simulink model "BBB_Gyro_Test_SFunction_Mask"  (R2013a)
settings: Solver=FixedStepDiscrete  StartTime=0.0  StopTime=inf  FixedStep=0.01  RelTol=1e-3
settings Model: SimulationMode=external  ExtModeTrigDuration=100  Creator=rdustinkahawita  LastModifiedBy=rdustinkahawita
settings OptimizationCC: OptimizeModelRefInitCode=on  LifeSpan=1
settings DebuggingCC: SolverPrmCheckMsg=none  StrictBusMsg=Warning
settings HardwareCC: ProdLargestAtomicInteger=Long  ProdLargestAtomicFloat=Double  ProdEndianess=LittleEndian  ProdHWDeviceType=ARM Compatible->ARM Cortex
settings RTWCC: SystemTargetFile=realtime.tlc  GenerateMakefile=off  TemplateMakefile=realtime.tmf  Description=Run on Target Hardware  RTWVerbose=off  ProcessScript=realtime_make_rtw_hook
settings STFCustomTargetCC: TargetLibSuffix=.a  GenerateSampleERTMain=on  ERTCustomFileBanners=on  SupportNonInlinedSFcns=off  SupportVariableSizeSignals=on  MATLABClassNameForMDSCustomization=Simulink.SoftwareTarget.ERTCustomization  SystemTargetFile=realtime.tlc
settings ERTTargetCC: ParMdlRefBuildCompliant=off  CompOptLevelCompliant=off  ConcurrentExecutionCompliant=off  CombineOutputUpdateFcns=off  ERTFirstTimeCompliant=off  SupportContinuousTime=on  SupportVariableSizeSignals=on  ModelStepFunctionPrototypeControlCompliant=off  CPPClassGenCompliant=off  ExtMode=on  ExtModeMexArgs='192.168.7.2' 0 17725  ERTSrcFileBannerTemplate=realtime_code_template.cgt  ERTHdrFileBannerTemplate=realtime_code_template.cgt  ERTDataSrcFileTemplate=realtime_code_template.cgt  ERTDataHdrFileTemplate=realtime_code_template.cgt  ERTCustomFileTemplate=realtime_file_process.tlc

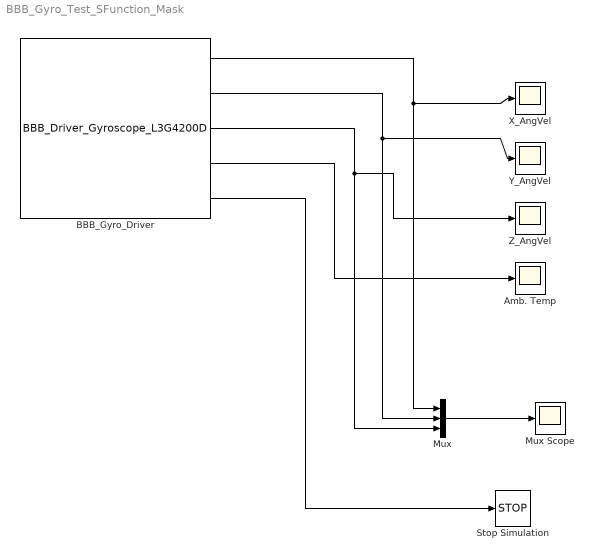
== system BBB_Gyro_Test_SFunction_Mask ==
  Amb. Temp : Scope
      settings: YMin=15.2  YMax=16.8  SaveName=ScopeData3
  "BBB_Gyro_Driver " : S-Function  FunctionName=BBB_Driver_Gyroscope_L3G4200D  Parameters=uint8(BBB_I2CBus),uint8(BBB_I2CAddress),uint8(BBB_GyroRange),uint8(BBB_DebugInfo)  SFunctionModules=BBB_Driver_Gyroscope_L3G4200D_wrapper  EnableBusSupport=off  mask(BLACKlink Album - BBB_Driver_Gyroscope_L3G4200D){BBB_I2CBus=BeagleBone Black I2C Channel 1, BBB_I2CAddress=Gyro Address: 0x068, BBB_GyroRange=Range: 250 deg/sec, BBB_DebugInfo=No Debug Info}
      mask prompts: BBB_I2CBus "Select I2C Channel on BeagleBoneBlack"; BBB_I2CAddress "Select I2C Device Address"; BBB_GyroRange "Select Gyro Range"; BBB_DebugInfo "Select Debug Info Level"
      mask help:
      | BeagleBone Black Driver Block:LG4200D Ultra-Stable 3-Axis Digital Gyroscope
      |
      | This
      mask Help:
      | Parameter Information:
      | 
      | I2C_Bus: Select the I2CBus on the BeagleBone Black to which the Gyroscope
      | device is connected to
      | 
      | Note on Block Validation:
      | - Hardware: BeagleBone Black (rev B)
      | - OS: Linux Ubuntu 13.10 (Saucy Salamander)
      | - GCC:4.8
      | - Linaro: 4.8.1
      | - Linux Kernel: Arm 3.8.13-bone32
      | - Arm Instruction Set Architechture: Armv71
      | 
      | 
      | 
      | 
      | Raw Version Data:
      | 
      | Linux arm 3.8.13-bone32 #1 SMP Fri Dec 13 20:05:25 UTC 2013 armv7l armv7l armv7l GNU/Linux
      | Using built-in specs.
      | COLLECT_GCC=gcc
      | COLLECT_LTO_WRAPPER=/usr/lib/gcc/arm-linux-gnueabihf/4.8/lto-wrapper
      | Target: arm-linux-gnueabihf
      | Configured with: ../src/configure -v --with-pkgversion='Ubuntu/Linaro 4.8.1-10ubuntu9' --with-bugurl=file:///usr/shar
      | e/doc/gcc-4.8/README.Bugs --enable-languages=c,c++,java,go,d,fortran,objc,obj-c++ --prefix=/usr --program-suffix=-4.8
      |  --enable-shared --enable-linker-build-id --libexecdir=/usr/lib --without-included-gettext --enable-threads=posix --w
      | ith-gxx-include-dir=/usr/include/c++/4.8 --libdir=/usr/lib --enable-nls --with-sysroot=/ --enable-clocale=gnu --enabl
      | e-libstdcxx-debug --enable-libstdcxx-time=yes --enable-gnu-unique-object --disable-libitm --disable-libquadmath --ena
      | ble-plugin --with-system-zlib --disable-browser-plugin --enable-java-awt=gtk --enable-gtk-cairo --with-java-home=/usr
      | /lib/jvm/java-1.5.0-gcj-4.8-armhf/jre --enable-java-home --with-jvm-root-dir=/usr/lib/jvm/java-1.5.0-gcj-4.8-armhf --
      | with-jvm-jar-dir=/usr/lib/jvm-exports/java-1.5.0-gcj-4.8-armhf --with-arch-directory=arm --with-ecj-jar=/usr/share/ja
      | va/eclipse-ecj.jar --enable-objc-gc --enable-multiarch --enable-multilib --disable-sjlj-exceptions --with-arch=armv7-
      | a --with-fpu=vfpv3-d16 --with-float=hard --with-mode=thumb --disable-werror --enable-checking=release --build=arm-lin
      | ux-gnueabihf --host=arm-linux-gnueabihf --target=arm-linux-gnueabihf
      | Thread model: posix
      | gcc version 4.8.1 (Ubuntu/Linaro 4.8.1-10ubuntu9)
      mask TypeOptions BBB_I2CBus: BeagleBone Black I2C Channel 1 | BeagleBone Black I2C Channel 2
      mask TypeOptions BBB_I2CAddress: Gyro Address: 0x068 | Gyro Address: 0x069
      mask TypeOptions BBB_GyroRange: Range: 250 deg/sec | Range: 500 deg/sec | Range: 2000 deg/sec
      mask TypeOptions BBB_DebugInfo: No Debug Info | Debug Level 0 - Basic Info Only | Debug Level 1 - Include Critical Info | Debug Level 2 - Include Diagnostics Info | Debug Level 3 - Include Program Flow Info | Debug Level 4 - Include Device Registery Read-Out | Debug Level 5 - + T.B.D.
      mask Display:
      | image(imread('BlackLink_Gyro.jpg'))
      | color('green');port_label('output',1,'outAngVel_X'), port_label('output',2,'outAngVel_Y'), port_label('output',3,'outAngVel_Z'), port_label('output',4,'outAmbTemp'), port_label('output',5,'outSimStop')
      | color('orange');
      | text(0,6,'BLACKlink')
  Mux : Mux  Inputs=3
  Mux Scope : Scope
      settings: ShowLegends=on  TimeRange=20  YMin=-150  YMax=175  SaveName=ScopeData4
  Stop Simulation : Stop
  X_AngVel : Scope
      settings: TimeRange=10  YMin=-300  YMax=250
  Y_AngVel : Scope
      settings: YMin=-300  YMax=300
  Z_AngVel : Scope
      settings: YMin=-300  YMax=250  SaveName=ScopeData2
  wires:
  Mux/1 -> Mux Scope/1
  "BBB_Gyro_Driver "/1 -> Mux/1, X_AngVel/1
  "BBB_Gyro_Driver "/2 -> Mux/2, Y_AngVel/1
  "BBB_Gyro_Driver "/3 -> Mux/3, Z_AngVel/1
  "BBB_Gyro_Driver "/4 -> Amb. Temp/1
  "BBB_Gyro_Driver "/5 -> Stop Simulation/1
